simulink model "dual500MHzPFB"  (Simulink 6.2)
settings: Solver=ode45  StartTime=0.0  StopTime=10000  RelTol=1e-3
libraries: xbsIndex_r3 x2070, casper_library x180, xps_library x12, gtkWave x5, gavrt_library x1
(part 9 of 20)

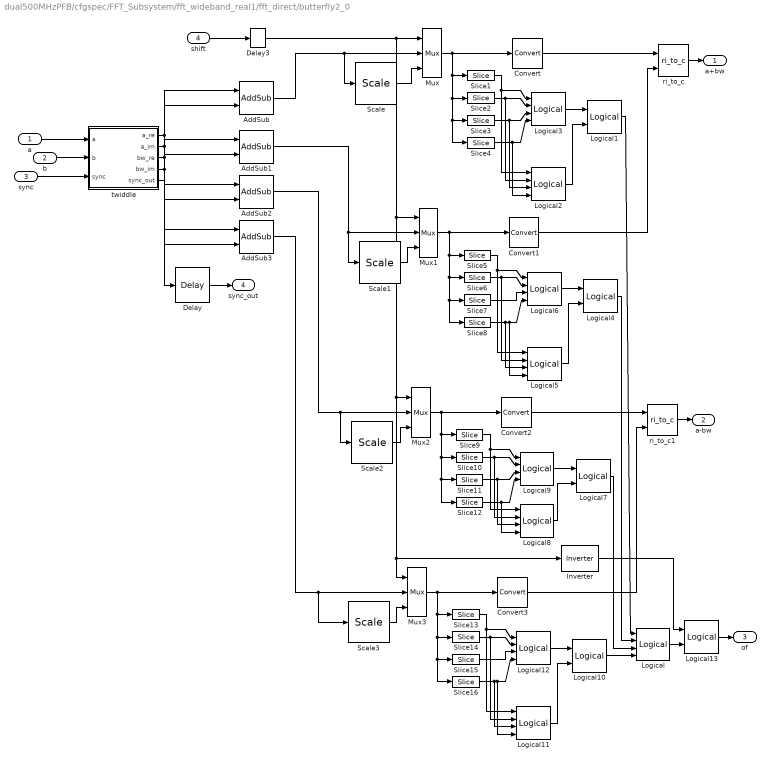
== system dual500MHzPFB/cfgspec/FFT_Subsystem/fft_wideband_real1/fft_direct/butterfly2_0 ==
  a : Inport  Port=1  LatchInput=off
  b : Inport  Port=2  LatchInput=off
  sync : Inport  Port=3  LatchInput=off
  shift : Inport  Port=4  LatchInput=off
  AddSub : xbsIndex_r3/AddSub  mode=Addition  precision=Full  arith_type=Unsigned  n_bits=8  bin_pt=2  quantization=Truncate  overflow=Wrap  latency=add_latency  explicit_period=off  period=1  use_carryin=off  use_carryout=off  en=off  dbl_ovrd=off  show_param=on  use_core=on  pipeline=on  use_rpm=on  gen_core=on
      settings: xl_area=[0, 0, 0, 0, 0, 0, 0]
  AddSub1 : xbsIndex_r3/AddSub  mode=Addition  precision=Full  arith_type=Unsigned  n_bits=8  bin_pt=2  quantization=Truncate  overflow=Wrap  latency=add_latency  explicit_period=off  period=1  use_carryin=off  use_carryout=off  en=off  dbl_ovrd=off  show_param=on  use_core=on  pipeline=on  use_rpm=on  gen_core=on
      settings: xl_area=[0, 0, 0, 0, 0, 0, 0]
  AddSub2 : xbsIndex_r3/AddSub  mode=Subtraction  precision=Full  arith_type=Unsigned  n_bits=8  bin_pt=2  quantization=Truncate  overflow=Wrap  latency=add_latency  explicit_period=off  period=1  use_carryin=off  use_carryout=off  en=off  dbl_ovrd=off  show_param=on  use_core=on  pipeline=on  use_rpm=on  gen_core=on
      settings: xl_area=[0, 0, 0, 0, 0, 0, 0]
  AddSub3 : xbsIndex_r3/AddSub  mode=Subtraction  precision=Full  arith_type=Unsigned  n_bits=8  bin_pt=2  quantization=Truncate  overflow=Wrap  latency=add_latency  explicit_period=off  period=1  use_carryin=off  use_carryout=off  en=off  dbl_ovrd=off  show_param=on  use_core=on  pipeline=on  use_rpm=on  gen_core=on
      settings: xl_area=[0, 0, 0, 0, 0, 0, 0]
  Convert{,1..3} (4 alike) : xbsIndex_r3/Convert  arith_type="Signed  (2's comp)"  n_bits=BitWidth  bin_pt=BitWidth-1  quantization=Truncate  overflow=Wrap  latency=add_latency  explicit_period=off  period=1  dbl_ovrd=off  show_param=off  inserted_by_tool=off  pipeline=off
      settings: xl_area=[0, 0, 0, 0, 0, 0, 0]
  Delay : xbsIndex_r3/Delay  latency=2 * add_latency + 1  reg_retiming=off  explicit_period=off  period=1  en=off  accept_only_valid=off  init_zero=on  dbl_ovrd=off  show_param=off
      settings: xl_area=[0, 0, 0, 0, 0, 0, 0]
  Delay3 : xbsIndex_r3/Delay  latency=1  reg_retiming=off  explicit_period=off  period=1  en=off  accept_only_valid=off  init_zero=on  dbl_ovrd=off  show_param=off
      settings: xl_area=[0, 0, 0, 0, 0, 0, 0]
  Inverter : xbsIndex_r3/Inverter  latency=0  explicit_period=off  period=1  en=off  dbl_ovrd=off  show_param=off
      settings: xl_area=[0, 0, 0, 0, 0, 0, 0]
  Logical : xbsIndex_r3/Logical  logical_function=OR  inputs=4  precision=Full  arith_type=Unsigned  n_bits=8  bin_pt=2  align_bp=on  latency=1  explicit_period=off  period=1  en=off  dbl_ovrd=off  show_param=off
      settings: xl_area=[0, 0, 0, 0, 0, 0, 0]
  Logical{1,4,7,10} (4 alike) : xbsIndex_r3/Logical  logical_function=OR  inputs=2  precision=Full  arith_type=Unsigned  n_bits=8  bin_pt=2  align_bp=off  latency=1  explicit_period=off  period=1  en=off  dbl_ovrd=off  show_param=off
      settings: xl_area=[0, 0, 0, 0, 0, 0, 0]
  Logical{2,5,8,11} (4 alike) : xbsIndex_r3/Logical  logical_function=NOR  inputs=4  precision=Full  arith_type=Unsigned  n_bits=8  bin_pt=2  align_bp=off  latency=1  explicit_period=off  period=1  en=off  dbl_ovrd=off  show_param=off
      settings: xl_area=[0, 0, 0, 0, 0, 0, 0]
  Logical{3,6,9,12} (4 alike) : xbsIndex_r3/Logical  logical_function=AND  inputs=4  precision=Full  arith_type=Unsigned  n_bits=8  bin_pt=2  align_bp=off  latency=1  explicit_period=off  period=1  en=off  dbl_ovrd=off  show_param=off
      settings: xl_area=[0, 0, 0, 0, 0, 0, 0]
  Logical13 : xbsIndex_r3/Logical  logical_function=AND  inputs=2  precision=Full  arith_type=Unsigned  n_bits=8  bin_pt=2  align_bp=off  latency=1  explicit_period=off  period=1  en=off  dbl_ovrd=off  show_param=off
      settings: xl_area=[0, 0, 0, 0, 0, 0, 0]
  Mux{,1..3} (4 alike) : xbsIndex_r3/Mux  inputs=2  precision=Full  arith_type="Signed  (2's comp)"  n_bits=8  bin_pt=2  quantization=Truncate  overflow=Wrap  latency=1  explicit_period=off  period=1  en=off  dbl_ovrd=off  show_param=off  mux_type=off  use_rpm=off  gen_core=off
      settings: xl_area=[0, 0, 0, 0, 0, 0, 0]
  Scale{,1..3} (4 alike) : xbsIndex_r3/Scale  scale_factor=-1  explicit_period=off  period=1  dbl_ovrd=off
  Slice{1,5,9,13} (4 alike) : xbsIndex_r3/Slice  mode=Upper Bit Location + Width  nbits=1  bit1=0  base1=MSB of Input  bit0=0  base0=LSB of Input  boolean_output=on  explicit_period=off  period=1  dbl_ovrd=off
  Slice{2,6,10,14} (4 alike) : xbsIndex_r3/Slice  mode=Upper Bit Location + Width  nbits=1  bit1=-1  base1=MSB of Input  bit0=0  base0=LSB of Input  boolean_output=on  explicit_period=off  period=1  dbl_ovrd=off
  Slice{3,7,11,15} (4 alike) : xbsIndex_r3/Slice  mode=Upper Bit Location + Width  nbits=1  bit1=-2  base1=MSB of Input  bit0=0  base0=LSB of Input  boolean_output=on  explicit_period=off  period=1  dbl_ovrd=off
  Slice{4,8,12,16} (4 alike) : xbsIndex_r3/Slice  mode=Upper Bit Location + Width  nbits=1  bit1=-3  base1=MSB of Input  bit0=0  base0=LSB of Input  boolean_output=on  explicit_period=off  period=1  dbl_ovrd=off
  ri_to_c : casper_library/Misc/ri_to_c
  ri_to_c1 : casper_library/Misc/ri_to_c
  twiddle : Subsystem  BlockChoice=twiddle_general_3mult
      link override twiddle_general_3mult: Coeffs="[1+0i               0.99998-0.0061359i       0.99992-0.012272i        0.99983-0.018407i         0.9997-0.024541i        0.99953-0.030675i        0.99932-0.036807i        0.99908-0.042938i         0.9988-0.049068i        0.99848-0.055195i        0.99812-0.061321i        0.99772-0.067444i        0.99729-0.073565i        0.99682-0.079682i        0.99631-0.085797i        0.99577-0.091909i        0.99518-0.098017i        0.99456-0.10412i         0.99391-0.11022i         0.99321-0.11632i         0.99248-0.12241i         0.99171-0.1285i           0.9909-0.13458i         0.99006-0.14066i         0.98918-0.14673i         0.98826-0.1528i           0.9873-0.15886i         0.98631-0.16491i         0.98528-0.17096i         0.98421-0.177i           0.98311-0.18304i         0.98196-0.18907i         0.98079-0.19509i         0.97957-0.2011i          0.97832-0.20711i         0.97703-0.21311i          0.9757-0.2191i          0.97434-0.22508i         0.97294-0.23106i          0.9715-0.23702i         0.97003-0.24298i         0.96852-0.24893i         0.96698-0.25487i         0.96539-0.26079i         0.96378-0.26671i         0.96212-0.27262i         0.96043-0.27852i          0.9587-0.28441i         0.95694-0.29028i         0.95514-0.29615i         0.95331-0.30201i         0.95144-0.30785i         0.94953-0.31368i         0.94759-0.3195i          0.94561-0.32531i         0.94359-0.33111i         0.94154-0.33689i         0.93946-0.34266i         0.93734-0.34842i         0.93518-0.35416i         0.93299-0.3599i          0.93077-0.36561i         0.92851-0.37132i         0.92621-0.37701i         0.92388-0.38268i         0.92151-0.38835i         0.91911-0.39399i         0.91668-0.39962i         0.91421-0.40524i         0.91171-0.41084i         0.90917-0.41643i          0.9066-0.422i           0.90399-0.42756i         0.90135-0.43309i         0.89867-0.43862i         0.89597-0.44412i         0.89322-0.44961i         0.89045-0.45508i         0.88764-0.46054i          0.8848-0.46598i         0.88192-0.4714i          0.87901-0.4768i          0.87607-0.48218i         0.87309-0.48755i         0.87009-0.4929i          0.86705-0.49823i         0.86397-0.50354i         0.86087-0.50883i         0.85773-0.5141i          0.85456-0.51936i         0.85136-0.52459i         0.84812-0.5298i          0.84485-0.535i           0.84155-0.54017i         0.83822-0.54532i         0.83486-0.55046i         0.83147-0.55557i         0.82805-0.56066i         0.82459-0.56573i          0.8211-0.57078i         0.81758-0.57581i         0.81404-0.58081i         0.81046-0.5858i          0.80685-0.59076i         0.80321-0.5957i          0.79954-0.60062i         0.79584-0.60551i         0.79211-0.61038i         0.78835-0.61523i         0.78456-0.62006i         0.78074-0.62486i         0.77689-0.62964i         0.77301-0.63439i          0.7691-0.63912i         0.76517-0.64383i          0.7612-0.64851i         0.75721-0.65317i         0.75319-0.65781i         0.74914-0.66242i         0.74506-0.667i           0.74095-0.67156i         0.73682-0.67609i         0.73265-0.6806i          0.72846-0.68508i         0.72425-0.68954i            0.72-0.69397i         0.71573-0.69838i         0.71143-0.70275i         0.70711-0.70711i         0.70275-0.71143i         0.69838-0.71573i         0.69397-0.72i            0.68954-0.72425i         0.68508-0.72846i          0.6806-0.73265i         0.67609-0.73682i         0.67156-0.74095i           0.667-0.74506i         0.66242-0.74914i         0.65781-0.75319i         0.65317-0.75721i         0.64851-0.7612i          0.64383-0.76517i         0.63912-0.7691i          0.63439-0.77301i         0.62964-0.77689i         0.62486-0.78074i         0.62006-0.78456i         0.61523-0.78835i         0.61038-0.79211i         0.60551-0.79584i         0.60062-0.79954i          0.5957-0.80321i         0.59076-0.80685i          0.5858-0.81046i         0.58081-0.81404i         0.57581-0.81758i         0.57078-0.8211i          0.56573-0.82459i         0.56066-0.82805i ...(+2392 chars)    ]"  StepPeriod=0  BitWidth=18  add_latency=3  mult_latency=3  bram_latency=2
      link override twiddle_general_3mult/coeff_gen: BlockChoice=br_coeff_gen
      link override twiddle_general_3mult/coeff_gen/br_coeff_gen: Coeffs=[1 2 3 4 5 6 7]  StepPeriod=4  BitWidth=10  bram_latency=6
      link override twiddle_general_3mult/coeff_gen/br_coeff_gen/ROM: distributed_mem=off
      link override twiddle_general_3mult/coeff_gen/br_coeff_gen/ROM1: distributed_mem=off
      link override twiddle_general_3mult/coeff_gen/static_coeff_gen/Constant: equ=P=C
      link override twiddle_general_3mult/coeff_gen/static_coeff_gen/Constant1: equ=P=C
      settings: AttributesFormatString=%<BlockChoice>  TemplateBlock=casper_library/FFTs/Twiddle/twiddle  MemberBlocks=twiddle_coeff_0,twiddle_coeff_1,twiddle_general_3mult,twiddle_general_4mult,twiddle_stage_2
  a+bw : Outport
  a-bw : Outport  Port=2
  of : Outport  Port=3
  sync_out : Outport  Port=4
  wires:
  Inverter/1 -> Logical13/1
  Logical13/1 -> of/1
  Logical/1 -> Logical13/2
  Delay3/1 -> Inverter/1, Mux3/1, Mux2/1, Mux1/1, Mux/1
  Logical7/1 -> Logical/3
  AddSub3/1 -> Scale3/1, Mux3/2
  Logical10/1 -> Logical/4
  Logical11/1 -> Logical10/2
  Logical12/1 -> Logical10/1
  Slice16/1 -> Logical11/3, Logical11/4, Logical12/4
  Slice15/1 -> Logical12/3
  Slice14/1 -> Logical11/2, Logical12/2
  Slice13/1 -> Logical11/1, Logical12/1
  Convert3/1 -> ri_to_c1/2
  Scale3/1 -> Mux3/3
  Mux3/1 -> Slice16/1, Slice15/1, Slice14/1, Slice13/1, Convert3/1
  AddSub2/1 -> Scale2/1, Mux2/2
  Logical8/1 -> Logical7/2
  Logical9/1 -> Logical7/1
  Slice12/1 -> Logical8/4, Logical9/4
  Slice11/1 -> Logical8/3, Logical9/3
  Slice10/1 -> Logical8/2, Logical9/2
  Slice9/1 -> Logical8/1, Logical9/1
  Convert2/1 -> ri_to_c1/1
  Scale2/1 -> Mux2/3
  Mux2/1 -> Slice12/1, Slice11/1, Slice10/1, Slice9/1, Convert2/1
  Logical4/1 -> Logical/2
  Logical5/1 -> Logical4/2
  Logical6/1 -> Logical4/1
  Slice8/1 -> Logical5/3, Logical5/4, Logical6/4
  Slice7/1 -> Logical6/3
  Slice6/1 -> Logical5/2, Logical6/2
  Slice5/1 -> Logical5/1, Logical6/1
  Convert1/1 -> ri_to_c/2
  Scale1/1 -> Mux1/3
  Mux1/1 -> Slice8/1, Slice7/1, Slice6/1, Slice5/1, Convert1/1
  Logical1/1 -> Logical/1
  Logical2/1 -> Logical1/2
  Logical3/1 -> Logical1/1
  Slice4/1 -> Logical2/4, Logical3/4
  Slice3/1 -> Logical2/3, Logical3/3
  Slice2/1 -> Logical2/2, Logical3/2
  Slice1/1 -> Logical2/1, Logical3/1
  Convert/1 -> ri_to_c/1
  Scale/1 -> Mux/3
  Mux/1 -> Slice4/1, Slice3/1, Slice2/1, Slice1/1, Convert/1
  shift/1 -> Delay3/1
  AddSub1/1 -> Scale1/1, Mux1/2
  AddSub/1 -> Scale/1, Mux/2
  Delay/1 -> sync_out/1
  ri_to_c1/1 -> a-bw/1
  ri_to_c/1 -> a+bw/1
  a/1 -> twiddle/1(a)
  b/1 -> twiddle/2(b)
  sync/1 -> twiddle/3(sync)
  twiddle/1(a_re) -> AddSub/1, AddSub2/1
  twiddle/2(a_im) -> AddSub1/1, AddSub3/1
  twiddle/3(bw_re) -> AddSub/2, AddSub2/2
  twiddle/4(bw_im) -> AddSub1/2, AddSub3/2
  twiddle/5(sync_out) -> Delay/1

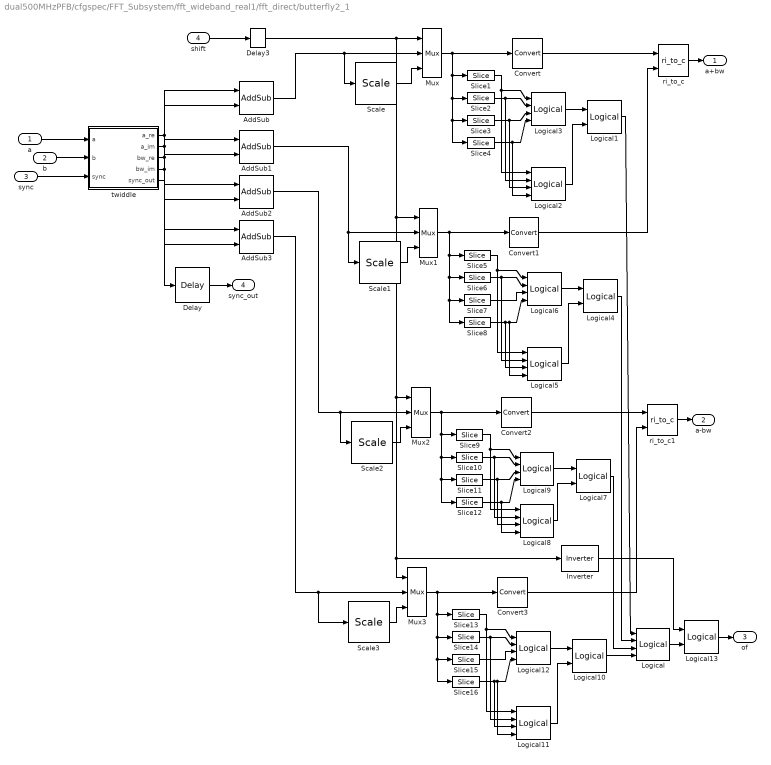
== system dual500MHzPFB/cfgspec/FFT_Subsystem/fft_wideband_real1/fft_direct/butterfly2_1 ==
  a : Inport  Port=1  LatchInput=off
  b : Inport  Port=2  LatchInput=off
  sync : Inport  Port=3  LatchInput=off
  shift : Inport  Port=4  LatchInput=off
  AddSub : xbsIndex_r3/AddSub  mode=Addition  precision=Full  arith_type=Unsigned  n_bits=8  bin_pt=2  quantization=Truncate  overflow=Wrap  latency=add_latency  explicit_period=off  period=1  use_carryin=off  use_carryout=off  en=off  dbl_ovrd=off  show_param=on  use_core=on  pipeline=on  use_rpm=on  gen_core=on
      settings: xl_area=[0, 0, 0, 0, 0, 0, 0]
  AddSub1 : xbsIndex_r3/AddSub  mode=Addition  precision=Full  arith_type=Unsigned  n_bits=8  bin_pt=2  quantization=Truncate  overflow=Wrap  latency=add_latency  explicit_period=off  period=1  use_carryin=off  use_carryout=off  en=off  dbl_ovrd=off  show_param=on  use_core=on  pipeline=on  use_rpm=on  gen_core=on
      settings: xl_area=[0, 0, 0, 0, 0, 0, 0]
  AddSub2 : xbsIndex_r3/AddSub  mode=Subtraction  precision=Full  arith_type=Unsigned  n_bits=8  bin_pt=2  quantization=Truncate  overflow=Wrap  latency=add_latency  explicit_period=off  period=1  use_carryin=off  use_carryout=off  en=off  dbl_ovrd=off  show_param=on  use_core=on  pipeline=on  use_rpm=on  gen_core=on
      settings: xl_area=[0, 0, 0, 0, 0, 0, 0]
  AddSub3 : xbsIndex_r3/AddSub  mode=Subtraction  precision=Full  arith_type=Unsigned  n_bits=8  bin_pt=2  quantization=Truncate  overflow=Wrap  latency=add_latency  explicit_period=off  period=1  use_carryin=off  use_carryout=off  en=off  dbl_ovrd=off  show_param=on  use_core=on  pipeline=on  use_rpm=on  gen_core=on
      settings: xl_area=[0, 0, 0, 0, 0, 0, 0]
  Convert{,1..3} (4 alike) : xbsIndex_r3/Convert  arith_type="Signed  (2's comp)"  n_bits=BitWidth  bin_pt=BitWidth-1  quantization=Truncate  overflow=Wrap  latency=add_latency  explicit_period=off  period=1  dbl_ovrd=off  show_param=off  inserted_by_tool=off  pipeline=off
      settings: xl_area=[0, 0, 0, 0, 0, 0, 0]
  Delay : xbsIndex_r3/Delay  latency=2 * add_latency + 1  reg_retiming=off  explicit_period=off  period=1  en=off  accept_only_valid=off  init_zero=on  dbl_ovrd=off  show_param=off
      settings: xl_area=[0, 0, 0, 0, 0, 0, 0]
  Delay3 : xbsIndex_r3/Delay  latency=1  reg_retiming=off  explicit_period=off  period=1  en=off  accept_only_valid=off  init_zero=on  dbl_ovrd=off  show_param=off
      settings: xl_area=[0, 0, 0, 0, 0, 0, 0]
  Inverter : xbsIndex_r3/Inverter  latency=0  explicit_period=off  period=1  en=off  dbl_ovrd=off  show_param=off
      settings: xl_area=[0, 0, 0, 0, 0, 0, 0]
  Logical : xbsIndex_r3/Logical  logical_function=OR  inputs=4  precision=Full  arith_type=Unsigned  n_bits=8  bin_pt=2  align_bp=on  latency=1  explicit_period=off  period=1  en=off  dbl_ovrd=off  show_param=off
      settings: xl_area=[0, 0, 0, 0, 0, 0, 0]
  Logical{1,4,7,10} (4 alike) : xbsIndex_r3/Logical  logical_function=OR  inputs=2  precision=Full  arith_type=Unsigned  n_bits=8  bin_pt=2  align_bp=off  latency=1  explicit_period=off  period=1  en=off  dbl_ovrd=off  show_param=off
      settings: xl_area=[0, 0, 0, 0, 0, 0, 0]
  Logical{2,5,8,11} (4 alike) : xbsIndex_r3/Logical  logical_function=NOR  inputs=4  precision=Full  arith_type=Unsigned  n_bits=8  bin_pt=2  align_bp=off  latency=1  explicit_period=off  period=1  en=off  dbl_ovrd=off  show_param=off
      settings: xl_area=[0, 0, 0, 0, 0, 0, 0]
  Logical{3,6,9,12} (4 alike) : xbsIndex_r3/Logical  logical_function=AND  inputs=4  precision=Full  arith_type=Unsigned  n_bits=8  bin_pt=2  align_bp=off  latency=1  explicit_period=off  period=1  en=off  dbl_ovrd=off  show_param=off
      settings: xl_area=[0, 0, 0, 0, 0, 0, 0]
  Logical13 : xbsIndex_r3/Logical  logical_function=AND  inputs=2  precision=Full  arith_type=Unsigned  n_bits=8  bin_pt=2  align_bp=off  latency=1  explicit_period=off  period=1  en=off  dbl_ovrd=off  show_param=off
      settings: xl_area=[0, 0, 0, 0, 0, 0, 0]
  Mux{,1..3} (4 alike) : xbsIndex_r3/Mux  inputs=2  precision=Full  arith_type="Signed  (2's comp)"  n_bits=8  bin_pt=2  quantization=Truncate  overflow=Wrap  latency=1  explicit_period=off  period=1  en=off  dbl_ovrd=off  show_param=off  mux_type=off  use_rpm=off  gen_core=off
      settings: xl_area=[0, 0, 0, 0, 0, 0, 0]
  Scale{,1..3} (4 alike) : xbsIndex_r3/Scale  scale_factor=-1  explicit_period=off  period=1  dbl_ovrd=off
  Slice{1,5,9,13} (4 alike) : xbsIndex_r3/Slice  mode=Upper Bit Location + Width  nbits=1  bit1=0  base1=MSB of Input  bit0=0  base0=LSB of Input  boolean_output=on  explicit_period=off  period=1  dbl_ovrd=off
  Slice{2,6,10,14} (4 alike) : xbsIndex_r3/Slice  mode=Upper Bit Location + Width  nbits=1  bit1=-1  base1=MSB of Input  bit0=0  base0=LSB of Input  boolean_output=on  explicit_period=off  period=1  dbl_ovrd=off
  Slice{3,7,11,15} (4 alike) : xbsIndex_r3/Slice  mode=Upper Bit Location + Width  nbits=1  bit1=-2  base1=MSB of Input  bit0=0  base0=LSB of Input  boolean_output=on  explicit_period=off  period=1  dbl_ovrd=off
  Slice{4,8,12,16} (4 alike) : xbsIndex_r3/Slice  mode=Upper Bit Location + Width  nbits=1  bit1=-3  base1=MSB of Input  bit0=0  base0=LSB of Input  boolean_output=on  explicit_period=off  period=1  dbl_ovrd=off
  ri_to_c : casper_library/Misc/ri_to_c
  ri_to_c1 : casper_library/Misc/ri_to_c
  twiddle : Subsystem  BlockChoice=twiddle_general_3mult
      link override twiddle_general_3mult: Coeffs="[6.1232e-017-1i            -0.0061359-0.99998i       -0.012272-0.99992i       -0.018407-0.99983i       -0.024541-0.9997i        -0.030675-0.99953i       -0.036807-0.99932i       -0.042938-0.99908i       -0.049068-0.9988i        -0.055195-0.99848i       -0.061321-0.99812i       -0.067444-0.99772i       -0.073565-0.99729i       -0.079682-0.99682i       -0.085797-0.99631i       -0.091909-0.99577i       -0.098017-0.99518i        -0.10412-0.99456i        -0.11022-0.99391i        -0.11632-0.99321i        -0.12241-0.99248i         -0.1285-0.99171i        -0.13458-0.9909i         -0.14066-0.99006i        -0.14673-0.98918i         -0.1528-0.98826i        -0.15886-0.9873i         -0.16491-0.98631i        -0.17096-0.98528i          -0.177-0.98421i        -0.18304-0.98311i        -0.18907-0.98196i        -0.19509-0.98079i         -0.2011-0.97957i        -0.20711-0.97832i        -0.21311-0.97703i         -0.2191-0.9757i         -0.22508-0.97434i        -0.23106-0.97294i        -0.23702-0.9715i         -0.24298-0.97003i        -0.24893-0.96852i        -0.25487-0.96698i        -0.26079-0.96539i        -0.26671-0.96378i        -0.27262-0.96212i        -0.27852-0.96043i        -0.28441-0.9587i         -0.29028-0.95694i        -0.29615-0.95514i        -0.30201-0.95331i        -0.30785-0.95144i        -0.31368-0.94953i         -0.3195-0.94759i        -0.32531-0.94561i        -0.33111-0.94359i        -0.33689-0.94154i        -0.34266-0.93946i        -0.34842-0.93734i        -0.35416-0.93518i         -0.3599-0.93299i        -0.36561-0.93077i        -0.37132-0.92851i        -0.37701-0.92621i        -0.38268-0.92388i        -0.38835-0.92151i        -0.39399-0.91911i        -0.39962-0.91668i        -0.40524-0.91421i        -0.41084-0.91171i        -0.41643-0.90917i          -0.422-0.9066i         -0.42756-0.90399i        -0.43309-0.90135i        -0.43862-0.89867i        -0.44412-0.89597i        -0.44961-0.89322i        -0.45508-0.89045i        -0.46054-0.88764i        -0.46598-0.8848i          -0.4714-0.88192i         -0.4768-0.87901i        -0.48218-0.87607i        -0.48755-0.87309i         -0.4929-0.87009i        -0.49823-0.86705i        -0.50354-0.86397i        -0.50883-0.86087i         -0.5141-0.85773i        -0.51936-0.85456i        -0.52459-0.85136i         -0.5298-0.84812i          -0.535-0.84485i        -0.54017-0.84155i        -0.54532-0.83822i        -0.55046-0.83486i        -0.55557-0.83147i        -0.56066-0.82805i        -0.56573-0.82459i        -0.57078-0.8211i         -0.57581-0.81758i        -0.58081-0.81404i         -0.5858-0.81046i        -0.59076-0.80685i         -0.5957-0.80321i        -0.60062-0.79954i        -0.60551-0.79584i        -0.61038-0.79211i        -0.61523-0.78835i        -0.62006-0.78456i        -0.62486-0.78074i        -0.62964-0.77689i        -0.63439-0.77301i        -0.63912-0.7691i         -0.64383-0.76517i        -0.64851-0.7612i         -0.65317-0.75721i        -0.65781-0.75319i        -0.66242-0.74914i          -0.667-0.74506i        -0.67156-0.74095i        -0.67609-0.73682i         -0.6806-0.73265i        -0.68508-0.72846i        -0.68954-0.72425i        -0.69397-0.72i           -0.69838-0.71573i        -0.70275-0.71143i        -0.70711-0.70711i        -0.71143-0.70275i        -0.71573-0.69838i           -0.72-0.69397i        -0.72425-0.68954i        -0.72846-0.68508i        -0.73265-0.6806i         -0.73682-0.67609i        -0.74095-0.67156i        -0.74506-0.667i          -0.74914-0.66242i        -0.75319-0.65781i        -0.75721-0.65317i         -0.7612-0.64851i        -0.76517-0.64383i         -0.7691-0.63912i        -0.77301-0.63439i        -0.77689-0.62964i        -0.78074-0.62486i        -0.78456-0.62006i        -0.78835-0.61523i        -0.79211-0.61038i        -0.79584-0.60551i        -0.79954-0.60062i        -0.80321-0.5957i         -0.80685-0.59076i        -0.81046-0.5858i         -0.81404-0.58081i        -0.81758-0.57581i         -0.8211-0.57078i        -0.82459-0.56573i        -0.82805-0.56066i ...(+2399 chars)  ]"  StepPeriod=0  BitWidth=18  add_latency=3  mult_latency=3  bram_latency=2
      link override twiddle_general_3mult/coeff_gen: BlockChoice=br_coeff_gen
      link override twiddle_general_3mult/coeff_gen/br_coeff_gen: Coeffs=[1 2 3 4 5 6 7]  StepPeriod=4  BitWidth=10  bram_latency=6
      link override twiddle_general_3mult/coeff_gen/br_coeff_gen/ROM: distributed_mem=off
      link override twiddle_general_3mult/coeff_gen/br_coeff_gen/ROM1: distributed_mem=off
      link override twiddle_general_3mult/coeff_gen/static_coeff_gen/Constant: equ=P=C
      link override twiddle_general_3mult/coeff_gen/static_coeff_gen/Constant1: equ=P=C
      settings: AttributesFormatString=%<BlockChoice>  TemplateBlock=casper_library/FFTs/Twiddle/twiddle  MemberBlocks=twiddle_coeff_0,twiddle_coeff_1,twiddle_general_3mult,twiddle_general_4mult,twiddle_stage_2
  a+bw : Outport
  a-bw : Outport  Port=2
  of : Outport  Port=3
  sync_out : Outport  Port=4
  wires:
  Inverter/1 -> Logical13/1
  Logical13/1 -> of/1
  Logical/1 -> Logical13/2
  Delay3/1 -> Inverter/1, Mux3/1, Mux2/1, Mux1/1, Mux/1
  Logical7/1 -> Logical/3
  AddSub3/1 -> Scale3/1, Mux3/2
  Logical10/1 -> Logical/4
  Logical11/1 -> Logical10/2
  Logical12/1 -> Logical10/1
  Slice16/1 -> Logical11/3, Logical11/4, Logical12/4
  Slice15/1 -> Logical12/3
  Slice14/1 -> Logical11/2, Logical12/2
  Slice13/1 -> Logical11/1, Logical12/1
  Convert3/1 -> ri_to_c1/2
  Scale3/1 -> Mux3/3
  Mux3/1 -> Slice16/1, Slice15/1, Slice14/1, Slice13/1, Convert3/1
  AddSub2/1 -> Scale2/1, Mux2/2
  Logical8/1 -> Logical7/2
  Logical9/1 -> Logical7/1
  Slice12/1 -> Logical8/4, Logical9/4
  Slice11/1 -> Logical8/3, Logical9/3
  Slice10/1 -> Logical8/2, Logical9/2
  Slice9/1 -> Logical8/1, Logical9/1
  Convert2/1 -> ri_to_c1/1
  Scale2/1 -> Mux2/3
  Mux2/1 -> Slice12/1, Slice11/1, Slice10/1, Slice9/1, Convert2/1
  Logical4/1 -> Logical/2
  Logical5/1 -> Logical4/2
  Logical6/1 -> Logical4/1
  Slice8/1 -> Logical5/3, Logical5/4, Logical6/4
  Slice7/1 -> Logical6/3
  Slice6/1 -> Logical5/2, Logical6/2
  Slice5/1 -> Logical5/1, Logical6/1
  Convert1/1 -> ri_to_c/2
  Scale1/1 -> Mux1/3
  Mux1/1 -> Slice8/1, Slice7/1, Slice6/1, Slice5/1, Convert1/1
  Logical1/1 -> Logical/1
  Logical2/1 -> Logical1/2
  Logical3/1 -> Logical1/1
  Slice4/1 -> Logical2/4, Logical3/4
  Slice3/1 -> Logical2/3, Logical3/3
  Slice2/1 -> Logical2/2, Logical3/2
  Slice1/1 -> Logical2/1, Logical3/1
  Convert/1 -> ri_to_c/1
  Scale/1 -> Mux/3
  Mux/1 -> Slice4/1, Slice3/1, Slice2/1, Slice1/1, Convert/1
  shift/1 -> Delay3/1
  AddSub1/1 -> Scale1/1, Mux1/2
  AddSub/1 -> Scale/1, Mux/2
  Delay/1 -> sync_out/1
  ri_to_c1/1 -> a-bw/1
  ri_to_c/1 -> a+bw/1
  a/1 -> twiddle/1(a)
  b/1 -> twiddle/2(b)
  sync/1 -> twiddle/3(sync)
  twiddle/1(a_re) -> AddSub/1, AddSub2/1
  twiddle/2(a_im) -> AddSub1/1, AddSub3/1
  twiddle/3(bw_re) -> AddSub/2, AddSub2/2
  twiddle/4(bw_im) -> AddSub1/2, AddSub3/2
  twiddle/5(sync_out) -> Delay/1

== system dual500MHzPFB/cfgspec/FFT_Subsystem/fft_wideband_real1/fft_unscrambler/reorder ==
  sync : Inport  Port=1  LatchInput=off
  en : Inport  Port=2  LatchInput=off
  din0 : Inport  Port=3  LatchInput=off
  din1 : Inport  Port=4  LatchInput=off
  Counter : xbsIndex_r3/Counter  cnt_type=Count Limited  n_bits=9  bin_pt=0  arith_type=Unsigned  start_count=0  cnt_to=511  cnt_by_val=1  operation=Up  explicit_period=off  period=1  load_pin=off  rst=on  en=on  dbl_ovrd=off  show_param=off  use_rpm=on  gen_core=off
      settings: xl_area=[0, 0, 0, 0, 0, 0, 0]
  Slice1 : xbsIndex_r3/Slice  mode=Upper Bit Location + Width  nbits=1  bit1=0  base1=MSB of Input  bit0=0  base0=LSB of Input  boolean_output=off  explicit_period=off  period=1  dbl_ovrd=off
  Slice2 : xbsIndex_r3/Slice  mode=Lower Bit Location + Width  nbits=8  bit1=0  base1=MSB of Input  bit0=0  base0=LSB of Input  boolean_output=off  explicit_period=off  period=1  dbl_ovrd=off
  dbl_buffer0 : casper_library/Reorder/dbl_buffer  depth=256  latency=2
  dbl_buffer1 : casper_library/Reorder/dbl_buffer  depth=256  latency=2
  delay_d0 : xbsIndex_r3/Delay  latency=2  reg_retiming=off  explicit_period=off  period=1  en=off  accept_only_valid=off  init_zero=on  dbl_ovrd=off  show_param=off
      settings: xl_area=[0, 0, 0, 0, 0, 0, 0]
  delay_din0 : xbsIndex_r3/Delay  latency=2  reg_retiming=off  explicit_period=off  period=1  en=off  accept_only_valid=off  init_zero=on  dbl_ovrd=off  show_param=off
      settings: xl_area=[0, 0, 0, 0, 0, 0, 0]
  delay_din1 : xbsIndex_r3/Delay  latency=2  reg_retiming=off  explicit_period=off  period=1  en=off  accept_only_valid=off  init_zero=on  dbl_ovrd=off  show_param=off
      settings: xl_area=[0, 0, 0, 0, 0, 0, 0]
  delay_sel : xbsIndex_r3/Delay  latency=2  reg_retiming=off  explicit_period=off  period=1  en=off  accept_only_valid=off  init_zero=on  dbl_ovrd=off  show_param=off
      settings: xl_area=[0, 0, 0, 0, 0, 0, 0]
  delay_valid : xbsIndex_r3/Delay  latency=4  reg_retiming=off  explicit_period=off  period=1  en=off  accept_only_valid=off  init_zero=on  dbl_ovrd=off  show_param=off
      settings: xl_area=[0, 0, 0, 0, 0, 0, 0]
  delay_we : xbsIndex_r3/Delay  latency=2  reg_retiming=off  explicit_period=off  period=1  en=off  accept_only_valid=off  init_zero=on  dbl_ovrd=off  show_param=off
      settings: xl_area=[0, 0, 0, 0, 0, 0, 0]
  map1 : xbsIndex_r3/ROM  depth=256  initVector=[0 2 4 6 8 10 12 14 16 18 20 22 24 26 28 30 32 34 36 38 40 42 44 46 48 50 52 54 56 58 60 62 64 66 68 70 72 74 76 78 80 82 84 86 88 90 92 94 96 98 100 102 104 106 108 110 112 114 116 118 120 122 124 126 128 130 132 134 136 138 140 142 144 146 148 150 152 154 156 158 160 162 164 166 168 170 172 174 176 178 180 182 184 186 188 190 192 194 196 198 200 202 204 206 208 210 212 214 216 218 220 222 224 226 228 230 232 234 236 238 240 242 244 246 248 250 252 254 1 3 5 7 9 11 13 15 17 19 21 23 25 27 29 31 33 35 37 39 41 43 45 47 49 51 53 55 57 59 61 63 65 67 69 71 73 75 77 79 81 83 85 87 89 91 93 95 97 99 101 103 105 107 109 111 113 115 117 119 121 123 125 127 129 131 133 135 137 139 141 143 145 147 149 151 153 155 157 159 161 163 165 167 169 171 173 175 177 179 181 183 185 187 189 191 193 195 197 199 201 203 205 207 209 211 213 215 217 219 221 223 225 227 229 231 233 235 237 239 241 243 245 247 249 251 253 255]  arith_type=Unsigned  n_bits=8  bin_pt=0  latency=2  init_zero=on  explicit_period=off  period=1  rst=off  init_reg=0  en=off  dbl_ovrd=off  show_param=off  distributed_mem=on  use_rpm=off  gen_core=off
      settings: xl_area=[0, 0, 0, 0, 0, 0, 0]
  post_sync_delay : xbsIndex_r3/Delay  latency=4  reg_retiming=off  explicit_period=off  period=1  en=off  accept_only_valid=off  init_zero=on  dbl_ovrd=off  show_param=off
      settings: xl_area=[0, 0, 0, 0, 0, 0, 0]
  pre_sync_delay : xbsIndex_r3/Delay  latency=2  reg_retiming=off  explicit_period=off  period=1  en=off  accept_only_valid=off  init_zero=on  dbl_ovrd=off  show_param=off
      settings: xl_area=[0, 0, 0, 0, 0, 0, 0]
  sync_delay_en : casper_library/Delays/sync_delay_en  DelayLen=256
      link override Constant: equ=P=C
      link override Constant1: equ=P=C
      link override Constant2: equ=P=C
      link override Constant3: equ=P=C
  sync_out : Outport
  valid : Outport  Port=2
  dout0 : Outport  Port=3
  dout1 : Outport  Port=4
  wires:
  sync/1 -> Counter/1, pre_sync_delay/1
  en/1 -> Counter/2, sync_delay_en/2, delay_we/1
  Counter/1 -> Slice1/1, Slice2/1
  Slice1/1 -> delay_sel/1
  Slice2/1 -> delay_d0/1, map1/1
  pre_sync_delay/1 -> sync_delay_en/1
  sync_delay_en/1 -> post_sync_delay/1
  post_sync_delay/1 -> sync_out/1
  delay_we/1 -> delay_valid/1, dbl_buffer0/5, dbl_buffer1/5
  delay_valid/1 -> valid/1
  delay_d0/1 -> dbl_buffer0/2, dbl_buffer1/2
  map1/1 -> dbl_buffer0/3, dbl_buffer1/3
  delay_sel/1 -> dbl_buffer0/1, dbl_buffer1/1
  din0/1 -> delay_din0/1
  delay_din0/1 -> dbl_buffer0/4
  dbl_buffer0/1 -> dout0/1
  din1/1 -> delay_din1/1
  delay_din1/1 -> dbl_buffer1/4
  dbl_buffer1/1 -> dout1/1

== system dual500MHzPFB/cfgspec/FFT_Subsystem/fft_wideband_real1/fft_unscrambler/square_transposer ==
  sync : Inport  Port=1  LatchInput=off
  In1 : Inport  Port=2  LatchInput=off
  In2 : Inport  Port=3  LatchInput=off
  Delayb1 : xbsIndex_r3/Delay  latency=1  reg_retiming=off  explicit_period=off  period=1  en=off  accept_only_valid=off  init_zero=on  dbl_ovrd=off  show_param=off
      settings: xl_area=[0, 0, 0, 0, 0, 0, 0]
  Delayb2 : xbsIndex_r3/Delay  latency=0  reg_retiming=off  explicit_period=off  period=1  en=off  accept_only_valid=off  init_zero=on  dbl_ovrd=off  show_param=off
      settings: xl_area=[0, 0, 0, 0, 0, 0, 0]
  Delayf1 : xbsIndex_r3/Delay  latency=0  reg_retiming=off  explicit_period=off  period=1  en=off  accept_only_valid=off  init_zero=on  dbl_ovrd=off  show_param=off
      settings: xl_area=[0, 0, 0, 0, 0, 0, 0]
  Delayf2 : xbsIndex_r3/Delay  latency=1  reg_retiming=off  explicit_period=off  period=1  en=off  accept_only_valid=off  init_zero=on  dbl_ovrd=off  show_param=off
      settings: xl_area=[0, 0, 0, 0, 0, 0, 0]
  barrel_switcher : Subsystem  AncestorBlock=casper_library/Reorder/barrel_switcher  mask(barrel_switcher){n_inputs=1}
      mask prompts: n_inputs "Number of Inputs: (2^?)"
      mask init:
      | barrel_switcher_init(gcb,...
      |     'n_inputs', n_inputs);
      settings: AttributesFormatString=n_inputs=1
  counter : xbsIndex_r3/Counter  cnt_type=Free Running  n_bits=n_inputs  bin_pt=0  arith_type=Unsigned  start_count=0  cnt_to=Inf  cnt_by_val=1  operation=Down  explicit_period=off  period=1  load_pin=off  rst=on  en=off  dbl_ovrd=off  show_param=off  use_rpm=on  gen_core=off
      settings: xl_area=[0, 0, 0, 0, 0, 0, 0]
  delay0 : xbsIndex_r3/Delay  latency=1  reg_retiming=off  explicit_period=off  period=1  en=off  accept_only_valid=off  init_zero=on  dbl_ovrd=off  show_param=off
      settings: xl_area=[0, 0, 0, 0, 0, 0, 0]
  sync_out : Outport
  Out1 : Outport  Port=2
  Out2 : Outport  Port=3
  wires:
  Delayb2/1 -> Out2/1
  barrel_switcher/3(Out2) -> Delayb2/1
  Delayf2/1 -> barrel_switcher/4(In2)
  In2/1 -> Delayf2/1
  Delayb1/1 -> Out1/1
  barrel_switcher/2(Out1) -> Delayb1/1
  Delayf1/1 -> barrel_switcher/3(In1)
  In1/1 -> Delayf1/1
  delay0/1 -> sync_out/1
  barrel_switcher/1(sync_out) -> delay0/1
  counter/1 -> barrel_switcher/1(sel)
  sync/1 -> barrel_switcher/2(sync_in), counter/1

== system dual500MHzPFB/cfgspec/PFB_Subsystem/pfb_fir_real/pol1_in1_first_tap/delay ==
  In1 : Inport  Port=1  LatchInput=off
  delay_bram : casper_library/Delays/delay_bram  DelayLen=2^(PFBSize-n_inputs)  bram_latency=bram_latency
  Out1 : Outport
  wires:
  In1/1 -> delay_bram/1
  delay_bram/1 -> Out1/1

== system dual500MHzPFB/cfgspec/PFB_Subsystem/pfb_fir_real/pol1_in1_first_tap/pfb_coeff_gen ==
  din : Inport  Port=1  LatchInput=off
  sync : Inport  Port=2  LatchInput=off
  Concat : xbsIndex_r3/Concat  num_inputs=2  explicit_period=off  period=1  dbl_ovrd=off
  Counter : xbsIndex_r3/Counter  cnt_type=Free Running  n_bits=8  bin_pt=0  arith_type=Unsigned  start_count=0  cnt_to=Inf  cnt_by_val=1  operation=Up  explicit_period=on  period=1  load_pin=off  rst=on  en=off  dbl_ovrd=off  show_param=off  use_rpm=on  gen_core=off
      settings: xl_area=[0, 0, 0, 0, 0, 0, 0]
  Delay : xbsIndex_r3/Delay  latency=bram_latency+1  reg_retiming=off  explicit_period=off  period=1  en=off  accept_only_valid=off  init_zero=on  dbl_ovrd=off  show_param=off
      settings: xl_area=[0, 0, 0, 0, 0, 0, 0]
  Delay1 : xbsIndex_r3/Delay  latency=3  reg_retiming=off  explicit_period=off  period=1  en=off  accept_only_valid=off  init_zero=on  dbl_ovrd=off  show_param=off
      settings: xl_area=[0, 0, 0, 0, 0, 0, 0]
  ROM1 : xbsIndex_r3/ROM  depth=256  initVector=[3.1185374660155e-018 0.000313853577146838 0.000630949867739494 0.000952101185429728 0.00127813150918155 0.00160987609990742 0.00194818110908897 0.00229390317955257 0.00264790903857445 0.00301107508349448 0.00338428696002226 0.00376843913342326 0.00416443445277708 0.00457318370850389 0.00499560518335912 0.00543262419710063 0.00588517264503594 0.00635418853066137 0.00684061549260819 0.00734540232611445 0.00786950249924483 0.00841387366408389 0.0089794771631314 0.00956727753113161 0.0101782419925713 0.010813339955084 0.0114735424990016 0.0121598218632949 0.0128731509281507 0.0136145026944319 0.014384849760272 0.0151851637950551 0.0160164150110379 0.0168795716328685 0.0177755993652613 0.0187054608590871 0.0196701151761411 0.0206705172528497 0.0217076173631834 0.0227823605810373 0.023895686242349 0.0250485274072193 0.0262418103223038 0.027476453883745 0.0287533691009129 0.0300734585612245 0.031437615896311 0.0328467252498039 0.0343016607470079 0.0358032859667318 0.0373524534155453 0.0389500040047317 0.0405967665302039 0.042293557155651 0.044041178899183 0.0458404211237378 0.0476920590315163 0.0495968531627079 0.0515555488987685 0.0535688759705108 0.0556375479712659 0.0577622618753727 0.0599436975622499 0.0621825173463032 0.0644793655129179 0.0668348678607861 0.0692496312508128 0.0717242431618448 0.0742592712534627 0.0768552629360733 0.0795127449485372 0.0822322229435622 0.0850141810810928 0.0878590816299174 0.0907673645777188 0.0937394472497809 0.0967757239365713 0.0998765655304047 0.103042319171399 0.106273307902919 0.109569830336718 0.112932160327956 0.116360546660299 0.119855212741273 0.123416356308059 0.127044149143908 0.13073873680534 0.134500238360297 0.138328746137415 0.142224325486561 0.146187014550802 0.15021682404994 0.154313737075755 0.158477708899094 0.162708666788946 0.167006509843603 0.171371108834052 0.175802306059696 0.180299915216515 0.184863721277773 0.189493480387363 0.194188919765877 0.198949737629496 0.203775603121767 0.208666156258342 0.213621007884754 0.218639739647272 0.22372190397691 0.228867024086619 0.234074593981714 0.239344078483567 0.244674913266598 0.250066504908579 0.255518230954276 0.261029439992432 0.266599451746097 0.272227557176302 0.277913018599066 0.283655069815719 0.289452916256518 0.29530573513754 0.301212675630786 0.307172859047495 0.313185379034582 0.31924930178417 0.325363666256144 0.331527484413666 0.33773974147157 0.343999396157563 0.350305380986143 0.356656602545143 0.363051941794802 0.369490254379254 0.375970370950336 0.382491097503579 0.389051215726279 0.395649483357505 0.402284634559911 0.40895538030322 0.415660408759225 0.422398385708151 0.429167954956233 0.435967738764334 0.44279633828744 0.449652334024857 0.456534286280925 0.46344073563607 0.470370203428 0.477321192242848 0.484292186416068 0.491281652542864 0.498288039997961 0.505309781464482 0.512345293471729 0.51939297694163 0.526451217743632 0.533518387257796 0.540592842945872 0.547672928930096 0.55475697657947 0.56184330510328 0.568930222151592 0.576016024422464 0.583098998275629 0.590177420352365 0.597249558201307 0.604313670909903 0.611368009741263 0.61841081877612 0.625440335559606 0.632454791752587 0.639452413787252 0.64643142352668 0.653390038928083 0.660326474709457 0.667238943019316 0.67412565410924 0.68098481700893 0.68781464020346 0.694613332312453 0.701379102770851 0.708110162510993 0.714804724645695 0.721461005152022 0.728077223555458 0.734651603614152 0.741182374002953 0.747667768996907 0.754106029153935 0.760495401996357 0.766834142690977 0.773120514727421 0.779352790594407 0.785529252453665 0.79164819281118 0.797707915185476 0.803706734772626 0.809642979107687 0.815514988722272 0.821321117797946 0.827059734815166 0.832729223197448 0.838327981950501 0.843854426296004 0.849306988299761 0.854684117493933 0.859984281493085 0.865205966603733 0.870347678427156 0.875407942455152 0.880385304658511 0.885278332067902 0.890085613346922 0.894805759357052 0.899437403714244 0.903979203336905 0.908429838985005 ...(+699 chars)]  arith_type="Signed  (2's comp)"  n_bits=8  bin_pt=7  latency=2  init_zero=on  explicit_period=off  period=1  rst=off  init_reg=0  en=off  dbl_ovrd=off  show_param=on  distributed_mem=off  use_rpm=on  gen_core=off
      settings: xl_area=[0, 0, 0, 0, 0, 0, 0]
  ROM2 : xbsIndex_r3/ROM  depth=256  initVector=[0.999999458258868 0.999931021245783 0.999743065596651 0.999435647723483 0.999008859879318 0.998462830120572 0.997797722254753 0.997013735773593 0.996111105771608 0.995090102850134 0.993951033006882 0.992694237511061 0.991320092764127 0.989829010146224 0.988221435848383 0.986497850690571 0.984658769925647 0.982704743029348 0.980636353476378 0.978454218502709 0.976158988854215 0.97375134852174 0.971232014462726 0.968601736309539 0.96586129606462 0.963011507782594 0.960053217239501 0.956987301589287 0.953814669007724 0.950536258323912 0.947153038639539 0.943666008936081 0.940076197670108 0.936384662356893 0.932592489142517 0.928700792364653 0.924710714102252 0.920623423714318 0.916440117367999 0.912162017556199 0.907790372604941 0.903326456170708 0.89877156672798 0.894127027047217 0.889394183663526 0.884574406336234 0.879669087499654 0.874679641705254 0.869607505055511 0.864454134629704 0.859221007901897 0.853909622151394 0.848521493865925 0.843058158137836 0.837521168053561 0.831912094076659 0.826232523424682 0.820484059440178 0.814668320956092 0.80878694165588 0.802841569428602 0.796833865719299 0.790765504874954 0.784638173486316 0.778453569725904 0.77221340268248 0.765919391692288 0.759573265667376 0.753176762421293 0.746731627992459 0.740239615965535 0.733702486791073 0.727122007103769 0.720499949039619 0.713838089552282 0.707138209728965 0.700402094106126 0.693631529985308 0.686828306749403 0.679994215179664 0.673131046773749 0.666240593065125 0.659324644944108 0.65238499198086 0.645423421750641 0.6384417191616 0.63144166578542 0.624425039191102 0.617393612282178 0.610349152637658 0.603293421856988 0.596228174909311 0.589155159487311 0.58207611536593 0.574992773766228 0.567906856724672 0.560820076468121 0.55373413479477 0.546650722461346 0.539571518576789 0.532498190002693 0.525432390760777 0.518375761447603 0.511329928656835 0.504296504409245 0.497277085590735 0.490273253398593 0.483286572796234 0.476318591976636 0.469370841834709 0.462444835448811 0.455542067571624 0.448664014130602 0.441812131738202 0.434987857212088 0.428192607105504 0.421427777248019 0.414694742296809 0.407994855298675 0.401329447262956 0.39469982674551 0.388107279443932 0.381553067804161 0.37503843063862 0.368564582756054 0.362132714603191 0.355743991918358 0.349399555397198 0.343100520370588 0.336847976494894 0.330642987454655 0.324486590677818 0.318379797063608 0.31232359072313 0.306318928732789 0.300366740900606 0.2944679295455 0.288623369289612 0.282833906863717 0.277100360925787 0.271423521892756 0.265804151785514 0.260242984087177 0.254740723614657 0.249298046403554 0.243915599606379 0.238594001404134 0.233333840931226 0.228135678213734 0.22300004412101 0.217927440330587 0.212918339306393 0.207973184290218 0.203092389306419 0.198276339179798 0.193525389566635 0.188839866998784 0.184220068940809 0.179666263860066 0.175178691309668 0.170757562024254 0.166403058028479 0.162115332758128 0.157894511193761 0.153740690006788 0.149653937717859 0.145634294867461 0.141681774198606 0.137796360851467 0.13397801256985 0.130226659919365 0.126542206517129 0.122924529272895 0.119373478641418 0.115888878885919 0.112470528352485 0.10911819975523 0.105831640472054 0.102610572850808 0.0994546945257127 0.0963636787438044 0.0933371747012584 0.0903748078893658 0.0874761804499801 0.0846408715402248 0.0818684377062569 0.0791584132658749 0.0765103106997557 0.0739236210511041 0.0713978143334908 0.0689323399466543 0.0665266271000393 0.0641800852438365 0.0618921045072929 0.0596620561440508 0.0574892929842778 0.0553731498933419 0.0533129442367877 0.0513079763513631 0.0493575300218483 0.0474608729634309 0.045617257309375 0.0438259201037253 0.0420860837987887 0.0403969567571315 0.0387577337578319 0.0371675965067231 0.0356257141503632 0.0341312437934655 0.0326833310195229 0.031281110414359 0.0299237060923366 0.0286102322249562 0.0273397935715735 0.0261114860119683 0.0249243970804927 0.0237776065015307 0.0226701867259983 0.0216012034686154 0.0205697162456796 0.019574778913074 ...(+681 chars)]  arith_type="Signed  (2's comp)"  n_bits=8  bin_pt=7  latency=2  init_zero=on  explicit_period=off  period=1  rst=off  init_reg=0  en=off  dbl_ovrd=off  show_param=on  distributed_mem=off  use_rpm=on  gen_core=off
      settings: xl_area=[0, 0, 0, 0, 0, 0, 0]
  Register : xbsIndex_r3/Register  init=0  reg_only_valid=off  explicit_period=off  period=1  rst=off  en=off  out_en=off  dbl_ovrd=off  show_param=off
      settings: xl_area=[0, 0, 0, 0, 0, 0, 0]
  Reinterpret1 : xbsIndex_r3/Reinterpret  force_arith_type=on  arith_type=Unsigned  force_bin_pt=on  bin_pt=0  force_valid=on
  Reinterpret2 : xbsIndex_r3/Reinterpret  force_arith_type=on  arith_type=Unsigned  force_bin_pt=on  bin_pt=0  force_valid=on
  dout : Outport
  sync_out : Outport  Port=2
  coeff : Outport  Port=3
  wires:
  din/1 -> Delay1/1
  Delay1/1 -> dout/1
  sync/1 -> Counter/1, Delay/1
  Delay/1 -> sync_out/1
  Concat/1 -> Register/1
  Register/1 -> coeff/1
  Counter/1 -> ROM1/1, ROM2/1
  ROM1/1 -> Reinterpret1/1
  Reinterpret1/1 -> Concat/1
  ROM2/1 -> Reinterpret2/1
  Reinterpret2/1 -> Concat/2
